simulink library "saturable_single_phase_transformer"  (R2025b)
settings: Solver=VariableStepAuto  StartTime=0.0  StopTime=10.0  RelTol=1e-3
libraries: nesl_utility x7, saturable_single_phase_transformer_2_lib x1
settings Model: Creator=dbagn  LastModifiedBy=dbagn

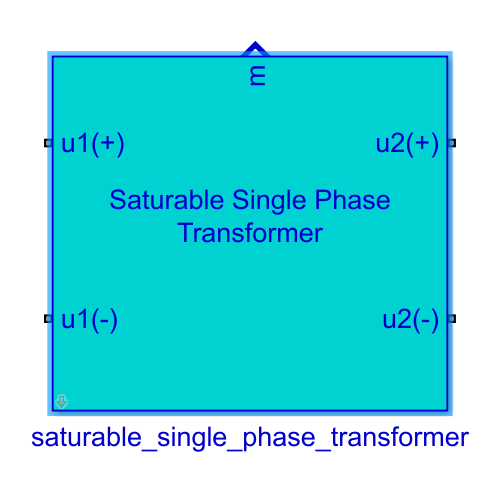
[thumbnail: Simulink's stored preview of the top-level diagram]
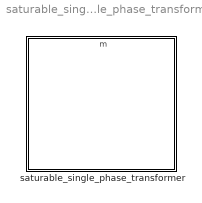
== system saturable_single_phase_transformer ==
  saturable_single_phase_transformer : Subsystem  mask{enable_sat_m=0, m1=43, m2=25, rd1_trafo=2e-3, rd2_trafo=2e-3, ld1_trafo=30e-6, ld2_trafo=30e-6, rfe_trafo=260, area_core=0.05, length_core=2.5, mu0=1.256637e-6, mur_m=20000, phi_sat_m=0.1}
      mask prompts: enable_sat_m "Enable Saturation"; m1 "N1"; m2 "N2"; rd1_trafo "rd1_trafo (Ohm)"; rd2_trafo "rd2_trafo (Ohm)"; ld1_trafo "ld1_trafo (H)"; ld2_trafo "ld2_trafo (H)"; rfe_trafo "rfe_trafo (Ohm)"; area_core "area_core (m^2)"; length_core "length_core (m)"; mu0 "mu0 (H/m)"; mur_m "mur"; phi_sat_m "phi_sat (Vs)"
      settings: PortSchema="{\"entries\":[{\"content\":{\"sides\":[{\"content\":{\"connectorIds\":[\"LConn1\",\"LConn2\"]},\"type\":\"ConnectorPlacement.EquallySpacedRectSide\",\"uuid\":\"cc5083b3-98b5-4a35-b4ef-aa8e070b6479\"},{\"content\":{\"connectorIds\":[\"RConn1\",\"RConn2\"],\"side\":\"RIGHT\"},\"type\":\"ConnectorPlacement.EquallySpacedRectSide\",\"uuid\":\"4f99e7ca-a3d1-47dd-a6e0-5288e9bf64fa\"},{\"content\":{\"connectorIds\":[\"Out1\"],\"side\":\"TOP\"},\"type\":\"ConnectorPlacement.EquallySpacedRectSide\",\"uuid\":\"04f8df7c-5b1b-4d7b-a78b-8566449322d4\"}]},\"type\":\"ConnectorPlacement.EquallySpacedConnector\",\"uuid\":\"acb55158-4a6e-48bb-9c2e-1677dfe1f617\"}],\"packageUris\":[\"http://schema.mathworks.com/mf0/Connector/R2020b\"],\"version\":\"1.0\"}"
      mask Display:
      | fprintf('Saturable Single Phase\nTransformer\n');
      | port_label('output', 1, 'm');
      | 
      | port_label('lconn', 1, 'u1(+)');
      | port_label('lconn', 2, 'u1(-)');
      | port_label('rconn', 1, 'u2(+)');
      | port_label('rconn', 2, 'u2(-)');

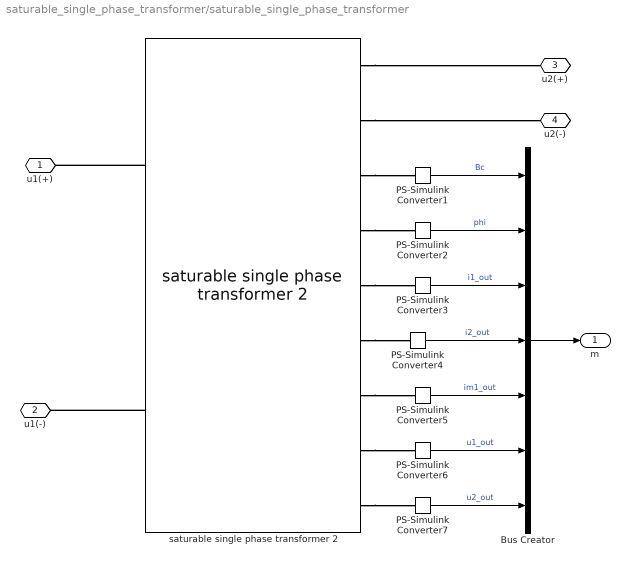
== system saturable_single_phase_transformer/saturable_single_phase_transformer ==
  Bus Creator : BusCreator  Inputs=7
  PS-Simulink Converter1 : nesl_utility/PS-Simulink Converter  PhysicalDomain=network_engine_domain  SubClassName=ps_output  LeftPortType=input  RightPortType=output  PseudoPeriodic=off  Frequencies=[]  VectorFormat=1-D array  Unit=Wb/m^2  AffineConversion=off
  PS-Simulink Converter2 : nesl_utility/PS-Simulink Converter  PhysicalDomain=network_engine_domain  SubClassName=ps_output  LeftPortType=input  RightPortType=output  PseudoPeriodic=off  Frequencies=[]  VectorFormat=1-D array  Unit=V*s  AffineConversion=off
  PS-Simulink Converter3 : nesl_utility/PS-Simulink Converter  PhysicalDomain=network_engine_domain  SubClassName=ps_output  LeftPortType=input  RightPortType=output  PseudoPeriodic=off  Frequencies=[]  VectorFormat=1-D array  Unit=A  AffineConversion=off
  PS-Simulink Converter4 : nesl_utility/PS-Simulink Converter  PhysicalDomain=network_engine_domain  SubClassName=ps_output  LeftPortType=input  RightPortType=output  PseudoPeriodic=off  Frequencies=[]  VectorFormat=1-D array  Unit=A  AffineConversion=off
  PS-Simulink Converter5 : nesl_utility/PS-Simulink Converter  PhysicalDomain=network_engine_domain  SubClassName=ps_output  LeftPortType=input  RightPortType=output  PseudoPeriodic=off  Frequencies=[]  VectorFormat=1-D array  Unit=A  AffineConversion=off
  PS-Simulink Converter6 : nesl_utility/PS-Simulink Converter  PhysicalDomain=network_engine_domain  SubClassName=ps_output  LeftPortType=input  RightPortType=output  PseudoPeriodic=off  Frequencies=[]  VectorFormat=1-D array  Unit=V  AffineConversion=off
  PS-Simulink Converter7 : nesl_utility/PS-Simulink Converter  PhysicalDomain=network_engine_domain  SubClassName=ps_output  LeftPortType=input  RightPortType=output  PseudoPeriodic=off  Frequencies=[]  VectorFormat=1-D array  Unit=V  AffineConversion=off
  saturable single phase transformer 2 : saturable_single_phase_transformer_2_lib/saturable single phase transformer 2  en_sat=enable_sat_m  n1=m1  n2=m2  core_area=area_core m^2  length_m=length_core m  Rd1=rd1_trafo Ohm  Rd2=rd2_trafo Ohm  Ld1=ld1_trafo H  Ld2=ld2_trafo H  Rfe=rfe_trafo Ohm  mu0=1.256637e-6 H/m  mur=mur_m  phi_sat=phi_sat_m V*s  phi_specify=off  phi_priority=None  phi=0 V*s  phi_nominal_specify=off  phi_nominal_value=1  phi_nominal_unit=V*s  i1_specify=off  i1_priority=High  i1=0 A  i1_nominal_specify=off  i1_nominal_value=1  i1_nominal_unit=A  i2_specify=off  i2_priority=High  i2=0 A  i2_nominal_specify=off  i2_nominal_value=1  i2_nominal_unit=A  im_specify=off  im_priority=None  im=0 A  im_nominal_specify=off  im_nominal_value=1  im_nominal_unit=A  ife_specify=off  ife_priority=None  ife=0 A  ife_nominal_specify=off  ife_nominal_value=1  ife_nominal_unit=A  u1_specify=off  u1_priority=None  u1=0 V  u1_nominal_specify=off  u1_nominal_value=1  u1_nominal_unit=V  u2_specify=off  u2_priority=None  u2=0 V  u2_nominal_specify=off  u2_nominal_value=1  u2_nominal_unit=V
      settings: InternalSimscapePortConfiguration="{\"Bottom\":[],\"Left\":[{\"id\":\"u1_p\",\"label\":\"u1(+)\",\"type\":\"foundation.electrical.electrical\"},{\"id\":\"u1_n\",\"label\":\"u1(-)\",\"type\":\"foundation.electrical.electrical\"}],\"Right\":[{\"id\":\"u2_p\",\"label\":\"u2(+)\",\"type\":\"foundation.electrical.electrical\"},{\"id\":\"u2_n\",\"label\":\"u2(-)\",\"type\":\"foundation.electrical.electrical\"},{\"id\":\"Bc\",\"label\":\"Bc\",\"type\":\"output\"},{\"id\":\"phi_out\",\"label\":\"phi\",\"type\":\"output\"},{\"id\":\"i1_out\",\"label\":\"i1_out\",\"type\":\"output\"},{\"id\":\"i2_out\",\"label\":\"i2_out\",\"type\":\"output\"},{\"id\":\"im_out\",\"label\":\"im_out\",\"type\":\"output\"},{\"id\":\"u1_out\",\"label\":\"u1_out\",\"type\":\"output\"},{\"id\":\"u2_out\",\"label\":\"u2_out\",\"type\":\"output\"}],\"Top\":[]}"
  u1(+) : PMIOPort  Side=Left
  u1(-) : PMIOPort  Port=2  Side=Left
  u2(+) : PMIOPort  Port=3  Side=Right
  u2(-) : PMIOPort  Port=4  Side=Right
  m : Outport
  wires:
  PS-Simulink Converter1/1 -> Bus Creator/1  "Bc"
  PS-Simulink Converter2/1 -> Bus Creator/2  "phi"
  Bus Creator/1 -> m/1
  PS-Simulink Converter3/1 -> Bus Creator/3  "i1_out"
  PS-Simulink Converter4/1 -> Bus Creator/4  "i2_out"
  PS-Simulink Converter5/1 -> Bus Creator/5  "im1_out"
  PS-Simulink Converter6/1 -> Bus Creator/6  "u1_out"
  PS-Simulink Converter7/1 -> Bus Creator/7  "u2_out"
  connections:
  saturable single phase transformer 2/RConn1 -- u2(+)/RConn1
  saturable single phase transformer 2/RConn4 -- PS-Simulink Converter2/LConn1
  saturable single phase transformer 2/RConn3 -- PS-Simulink Converter1/LConn1
  saturable single phase transformer 2/LConn1 -- u1(+)/RConn1
  saturable single phase transformer 2/LConn2 -- u1(-)/RConn1
  saturable single phase transformer 2/RConn2 -- u2(-)/RConn1
  saturable single phase transformer 2/RConn5 -- PS-Simulink Converter3/LConn1
  saturable single phase transformer 2/RConn6 -- PS-Simulink Converter4/LConn1
  saturable single phase transformer 2/RConn7 -- PS-Simulink Converter5/LConn1
  saturable single phase transformer 2/RConn8 -- PS-Simulink Converter6/LConn1
  saturable single phase transformer 2/RConn9 -- PS-Simulink Converter7/LConn1
